simulink model "A1MODEL_Synthetic_Inv_Resp_delay"  (R2019a)
settings: Solver=VariableStepAuto  StartTime=0  StopTime=20  RelTol=1e-3
values from neighbouring files (symbols this model uses):
  c = 1    [calc_nadir.m]    (also in calc_variables_block.m; graph_freq_SI.m; graph_freq_SI_normal.m = 0; graph_freq_fpr.m)
  ci = 0    [calc_nadir.m]    (also in calc_variables_block.m; graph_freq_SI.m = 1; graph_freq_SI_normal.m = 1; graph_freq_fpr.m)
  d = 0.2    [calc_nadir.m]    (also in calc_variables_block.m = 0.001)
  E_load = 0    [calc_nadir.m]    (also in calc_variables_block.m; graph_freq_SI.m; graph_freq_SI_normal.m; graph_freq_fpr.m)
  F = data1(7)    [calc_nadir.m]    (also in calc_variables_block.m; graph_freq_SI.m; graph_freq_SI_normal.m; graph_freq_fpr.m)
  H = data1(9)    [calc_nadir.m]    (also in calc_variables_block.m; graph_freq_SI.m; graph_freq_SI_normal.m; graph_freq_fpr.m)
  H_wt = 4.37    [calc_nadir.m]    (also in calc_variables_block.m; graph_freq_SI.m; graph_freq_SI_normal.m; graph_freq_fpr.m)
  J = 3.56    [calc_nadir.m]    (also in calc_variables_block.m; graph_freq_SI.m; graph_freq_SI_normal.m; graph_freq_fpr.m)
  Ki = 10    [calc_nadir.m]    (also in calc_variables_block.m; graph_freq_SI.m; graph_freq_SI_normal.m; graph_freq_fpr.m)
  n_wt = P_re*share_wt/1.5    [calc_nadir.m]    (also in calc_variables_block.m; graph_freq_SI.m = P_wt/1.5; graph_freq_SI_normal.m = 0.666666666667; graph_freq_fpr.m)
  P_wt = P_re*share_wt    [calc_nadir.m]    (also in calc_variables_block.m; graph_freq_SI.m; graph_freq_SI_normal.m; graph_freq_fpr.m)
  R = 0.05    [calc_nadir.m]    (also in calc_variables_block.m; graph_freq_SI.m; graph_freq_SI_normal.m; graph_freq_fpr.m)
  Sb = data1(1)    [calc_nadir.m]    (also in calc_variables_block.m; graph_freq_SI.m; graph_freq_SI_normal.m; graph_freq_fpr.m)
  T_1 = data1(2)    [calc_nadir.m]    (also in calc_variables_block.m; graph_freq_SI.m; graph_freq_SI_normal.m; graph_freq_fpr.m)
  T_2 = data1(3)    [calc_nadir.m]    (also in calc_variables_block.m; graph_freq_SI.m; graph_freq_SI_normal.m; graph_freq_fpr.m)
  T_3 = data1(4)    [calc_nadir.m]    (also in calc_variables_block.m; graph_freq_SI.m; graph_freq_SI_normal.m; graph_freq_fpr.m)
  T_4 = data1(5)    [calc_nadir.m]    (also in calc_variables_block.m; graph_freq_SI.m; graph_freq_SI_normal.m; graph_freq_fpr.m)
  T_5 = data1(6)    [calc_nadir.m]    (also in calc_variables_block.m; graph_freq_SI.m; graph_freq_SI_normal.m; graph_freq_fpr.m)
  T_wt = 1    [calc_nadir.m]    (also in calc_variables_block.m; graph_freq_SI.m; graph_freq_SI_normal.m; graph_freq_fpr.m)
  un = 0.4    [calc_nadir.m]    (also in calc_variables_block.m; graph_freq_SI.m; graph_freq_SI_normal.m = 0.15; graph_freq_fpr.m = 0.25)
libraries: simulink x1
settings Model: Creator=estuser04  LastModifiedBy=Alejandro
settings DataIOCC: ReturnWorkspaceOutputs=off
settings DebuggingCC: ArithmeticOperatorsInVariantConditions=warning

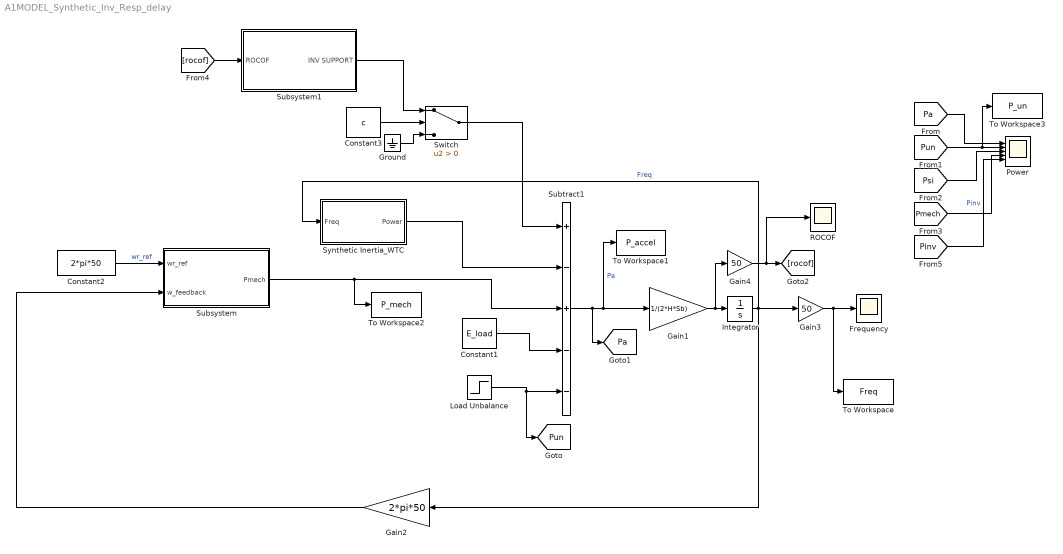
== system A1MODEL_Synthetic_Inv_Resp_delay ==
  Constant1 : Constant  Value=E_load
  Constant2 : Constant  Value=2*pi*50
  Constant3 : Constant  Value=c
  "Frequency " : Scope
  Gain1 : Gain  Gain=1/(2*H*Sb)
  Gain2 : Gain  Gain=2*pi*50
  Gain3 : Gain  Gain=50
  Gain4 : Gain  Gain=50
  Ground : Ground
  Integrator : Integrator  InitialCondition=1
  Load Unbalance : Step  Time=0  After=315*un  SampleTime=0
  Power : Scope  NumInputPorts=5
  ROCOF : Scope
  Subsystem : Subsystem
  Subsystem1 : Subsystem
  Subtract1 : Sum  Inputs=+-+--
  Switch : Switch  Criteria=u2 > Threshold
  "Synthetic Inertia_WTC " : Subsystem
  To Workspace : ToWorkspace  VariableName=Freq  SaveFormat=Timeseries  SampleTime=-1
  To Workspace1 : ToWorkspace  VariableName=P_accel  SaveFormat=Timeseries  SampleTime=-1
  To Workspace2 : ToWorkspace  VariableName=P_mech  SaveFormat=Timeseries  SampleTime=-1
  To Workspace3 : ToWorkspace  VariableName=P_un  SaveFormat=Timeseries  SampleTime=-1
  tag scope: Pa=global, Pun=global
  wires:
  Gain1/1 -> Gain4/1, Integrator/1
  Integrator/1 -> "Synthetic Inertia_WTC "/1(Freq), Gain3/1, Gain2/1  "Freq"
  Subtract1/1 -> [Pa], To Workspace1/1, Gain1/1  "Pa"
  Constant1/1 -> Subtract1/4
  Load Unbalance/1 -> Subtract1/5, [Pun]
  Gain3/1 -> To Workspace/1, "Frequency "/1
  Constant2/1 -> Subsystem/1(wr_ref)  "wr_ref"
  Gain2/1 -> Subsystem/2(w_feedback)
  Subsystem/1(Pmech) -> Subtract1/3, To Workspace2/1
  [Pa] -> Power/1
  [Pun] -> To Workspace3/1, Power/2
  [Psi] -> Power/3
  [Pmech] -> Power/4
  Switch/1 -> Subtract1/1
  Ground/1 -> Switch/3
  Constant3/1 -> Switch/2
  Gain4/1 -> ROCOF/1, [rocof]
  [rocof] -> Subsystem1/1(ROCOF)
  [Pinv] -> Power/5  "Pinv"
  "Synthetic Inertia_WTC "/1("Power ") -> Subtract1/2
  Subsystem1/1(INV SUPPORT) -> Switch/1

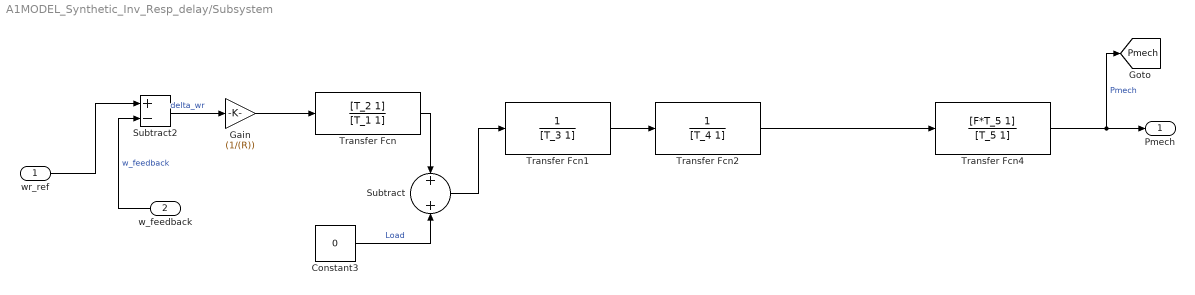
== system A1MODEL_Synthetic_Inv_Resp_delay/Subsystem ==
  wr_ref : Inport
  w_feedback : Inport  Port=2
  Constant3 : Constant  Value=0
  Gain : Gain  Gain=(1/(R))
  Subtract : Sum
  Subtract2 : Sum  Inputs=+-
  Transfer Fcn : TransferFcn  Numerator=[T_2 1]  Denominator=[T_1 1]
  Transfer Fcn1 : TransferFcn  Denominator=[T_3 1]
  Transfer Fcn2 : TransferFcn  Denominator=[T_4 1]
  Transfer Fcn4 : TransferFcn  Numerator=[F*T_5 1]  Denominator=[T_5 1]
  Pmech : Outport
  tag scope: Pmech=global
  wires:
  Constant3/1 -> Subtract/2  "Load"
  Transfer Fcn/1 -> Subtract/1
  Gain/1 -> Transfer Fcn/1
  Transfer Fcn2/1 -> Transfer Fcn4/1
  Subtract/1 -> Transfer Fcn1/1
  Subtract2/1 -> Gain/1  "delta_wr"
  w_feedback/1 -> Subtract2/2  "w_feedback"
  Transfer Fcn1/1 -> Transfer Fcn2/1
  wr_ref/1 -> Subtract2/1
  Transfer Fcn4/1 -> [Pmech], Pmech/1  "Pmech"

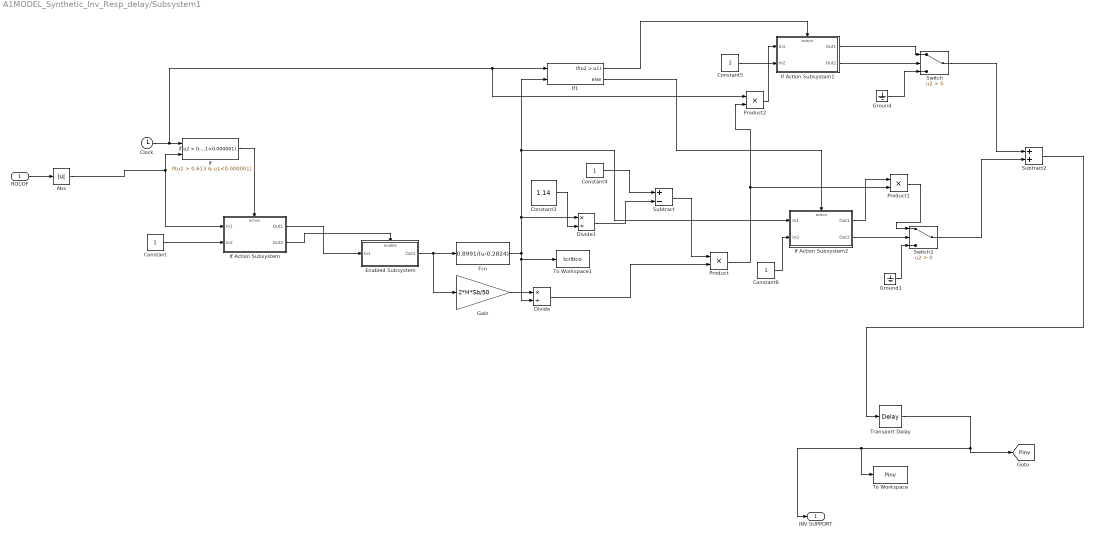
== system A1MODEL_Synthetic_Inv_Resp_delay/Subsystem1 ==
  ROCOF : Inport
  Abs : Abs  ZeroCross=off
  Clock : Clock
  Constant{,4..6} (4 alike) : Constant
  Constant3 : Constant  Value=1.14
  Divide : Product  Inputs=*/
  Divide1 : Product  Inputs=*/
  Enabled Subsystem : Subsystem  TreatAsAtomicUnit=on
  Fcn : Fcn  Expr=0.8991/(u-0.2824)
  Gain : Gain  Gain=2*H*Sb/50
  Ground : Ground
  Ground1 : Ground
  If : If  NumInputs=2  IfExpression=u2 > 0.613 & u1<0.000001  ShowElse=off
  If Action Subsystem : Subsystem  TreatAsAtomicUnit=on
  If Action Subsystem1 : Subsystem  TreatAsAtomicUnit=on
  If Action Subsystem2 : Subsystem  TreatAsAtomicUnit=on
  If1 : If  NumInputs=2  IfExpression=u2 > u1
  Product : Product
  Product1 : Product
  Product2 : Product
  Subtract : Sum  Inputs=+-
  Subtract2 : Sum
  Switch : Switch  Criteria=u2 > Threshold
  Switch1 : Switch  Criteria=u2 > Threshold
  To Workspace : ToWorkspace  VariableName=Pinv  SaveFormat=Timeseries  SampleTime=-1
  To Workspace1 : ToWorkspace  VariableName=tcritico  SaveFormat=Timeseries  SampleTime=-1
  Transport Delay : TransportDelay  DelayTime=d
  INV SUPPORT : Outport
  tag scope: Pinv=global
  wires:
  Switch1/1 -> Subtract2/2
  If Action Subsystem2/2(Out2) -> Switch1/2
  Divide/1 -> Product/2
  Product/1 -> Product1/2, Product2/2
  Constant4/1 -> Subtract/1
  Fcn/1 -> Divide/2, To Workspace1/1, If Action Subsystem2/1(In1), If1/2, Divide1/1
  If Action Subsystem/2(Out2) -> Enabled Subsystem/Enable
  Clock/1 -> Product2/1, If1/1, If/1
  Ground/1 -> Switch/3
  Divide1/1 -> Subtract/2
  Constant3/1 -> Divide1/2
  Enabled Subsystem/1(Out1) -> Gain/1, Fcn/1
  If Action Subsystem/1(Out1) -> Enabled Subsystem/1(In1)
  Subtract/1 -> Product/1
  If Action Subsystem1/2(Out2) -> Switch/2
  If1/1 -> If Action Subsystem1/Action
  Subtract2/1 -> Transport Delay/1
  Gain/1 -> Divide/1
  Ground1/1 -> Switch1/3
  If Action Subsystem2/1(Out1) -> Product1/1
  ROCOF/1 -> Abs/1
  Product1/1 -> Switch1/1
  If Action Subsystem1/1(Out1) -> Switch/1
  Constant6/1 -> If Action Subsystem2/2(In2)
  Constant5/1 -> If Action Subsystem1/2(In2)
  Switch/1 -> Subtract2/1
  Constant/1 -> If Action Subsystem/2(In2)
  Abs/1 -> If Action Subsystem/1(In1), If/2
  If1/2 -> If Action Subsystem2/Action
  Product2/1 -> If Action Subsystem1/1(In1)
  Transport Delay/1 -> [Pinv], To Workspace/1, INV SUPPORT/1
  If/1 -> If Action Subsystem/Action

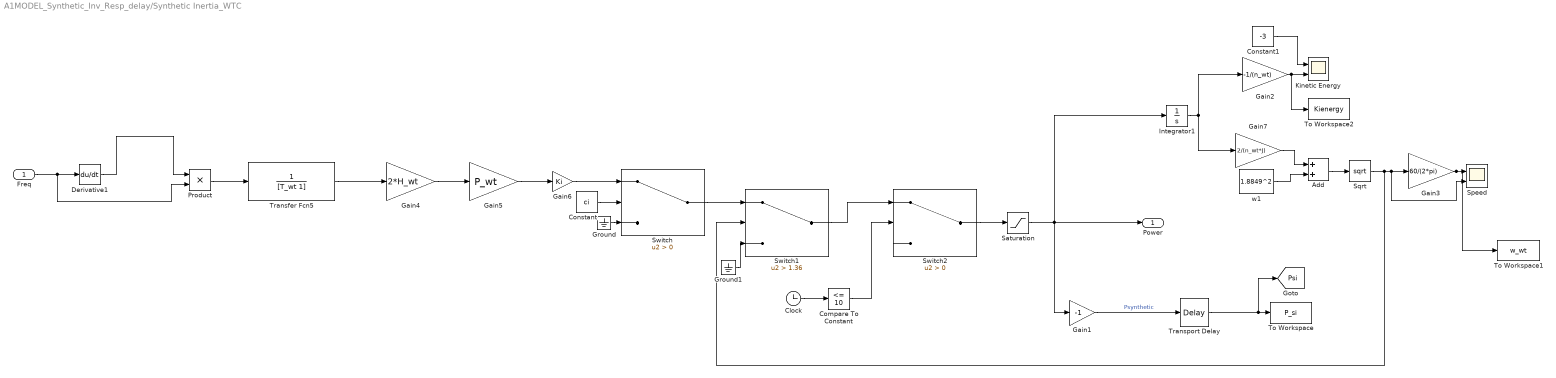
== system A1MODEL_Synthetic_Inv_Resp_delay/Synthetic Inertia_WTC  ==
  Freq : Inport
  Add : Sum
  Clock : Clock
  Compare To Constant : simulink/Logic and Bit Operations/Compare To Constant  relop=<=  const=10  OutDataTypeStr=boolean
  Constant : Constant  Value=ci
  Constant1 : Constant  Value=-3
  Derivative1 : Derivative
  Gain1 : Gain  Gain=-1
  Gain2 : Gain  Gain=-1/(n_wt)
  Gain3 : Gain  Gain=60/(2*pi)
  Gain4 : Gain  Gain=2*H_wt
  Gain5 : Gain  Gain=P_wt
  Gain6 : Gain  Gain=Ki
  Gain7 : Gain  Gain=2/(n_wt*J)
  Ground : Ground
  Ground1 : Ground
  Integrator1 : Integrator
  "Kinetic Energy " : Scope  NumInputPorts=2
  Product : Product
  Saturation : Saturate  UpperLimit=0  LowerLimit=-P_wt*0.10
  "Speed " : Scope  NumInputPorts=2
  Sqrt : Sqrt  SaturateOnIntegerOverflow=on
  Switch : Switch  Criteria=u2 > Threshold
  Switch1 : Switch  Criteria=u2 > Threshold  Threshold=1.36
  Switch2 : Switch  Criteria=u2 > Threshold
  To Workspace : ToWorkspace  VariableName=P_si  SaveFormat=Timeseries  SampleTime=-1
  To Workspace1 : ToWorkspace  VariableName=w_wt  SaveFormat=Timeseries  SampleTime=-1
  To Workspace2 : ToWorkspace  VariableName=Kienergy  SaveFormat=Timeseries  SampleTime=-1
  Transfer Fcn5 : TransferFcn  Denominator=[T_wt 1]
  Transport Delay : TransportDelay  DelayTime=d
  w1 : Constant  Value=1.8849^2
  "Power " : Outport
  tag scope: Psi=global
  wires:
  Gain5/1 -> Gain6/1
  Switch/1 -> Switch1/1
  Gain7/1 -> Add/1
  Gain4/1 -> Gain5/1
  Add/1 -> Sqrt/1
  Freq/1 -> Product/2, Derivative1/1
  w1/1 -> Add/2
  Product/1 -> Transfer Fcn5/1
  Transfer Fcn5/1 -> Gain4/1
  Constant/1 -> Switch/2
  Integrator1/1 -> Gain7/1, Gain2/1
  Gain6/1 -> Switch/1
  Ground/1 -> Switch/3
  Gain1/1 -> Transport Delay/1  "Psynthetic"
  Switch1/1 -> Switch2/1
  Sqrt/1 -> Switch1/2, "Speed "/2, Gain3/1
  Ground1/1 -> Switch1/3
  Gain2/1 -> To Workspace2/1, "Kinetic Energy "/2
  Constant1/1 -> "Kinetic Energy "/1
  Saturation/1 -> "Power "/1, Gain1/1, Integrator1/1
  Derivative1/1 -> Product/1
  Gain3/1 -> To Workspace1/1, "Speed "/1
  Clock/1 -> Compare To Constant/1
  Compare To Constant/1 -> Switch2/2
  Switch2/1 -> Saturation/1
  Transport Delay/1 -> [Psi], To Workspace/1

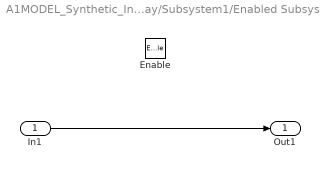
== system A1MODEL_Synthetic_Inv_Resp_delay/Subsystem1/Enabled Subsystem ==
  In1 : Inport
  Enable : EnablePort
  Out1 : Outport
  wires:
  In1/1 -> Out1/1

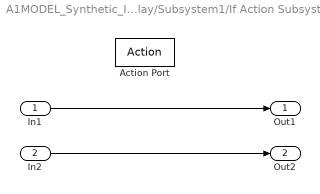
== system A1MODEL_Synthetic_Inv_Resp_delay/Subsystem1/If Action Subsystem ==
  In1 : Inport
  In2 : Inport  Port=2
  Action Port : ActionPort  ActionPortLabel=if(u2 > 0.613 & u1<0.000001)
  Out1 : Outport
  Out2 : Outport  Port=2
  wires:
  In1/1 -> Out1/1
  In2/1 -> Out2/1

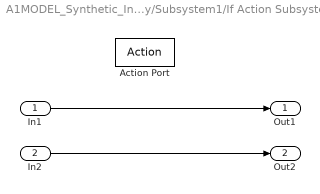
== system A1MODEL_Synthetic_Inv_Resp_delay/Subsystem1/If Action Subsystem1 ==
  In1 : Inport
  In2 : Inport  Port=2
  Action Port : ActionPort  ActionPortLabel=if(u2 > u1)
  Out1 : Outport  OutputWhenDisabled=reset  InitialOutput=0
  Out2 : Outport  Port=2  OutputWhenDisabled=reset  InitialOutput=0
  wires:
  In1/1 -> Out1/1
  In2/1 -> Out2/1

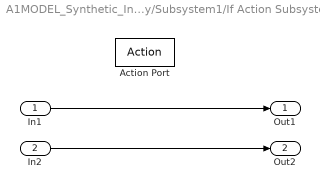
== system A1MODEL_Synthetic_Inv_Resp_delay/Subsystem1/If Action Subsystem2 ==
  In1 : Inport
  In2 : Inport  Port=2
  Action Port : ActionPort  ActionPortLabel=else
  Out1 : Outport  OutputWhenDisabled=reset  InitialOutput=0
  Out2 : Outport  Port=2  InitialOutput=0
  wires:
  In1/1 -> Out1/1
  In2/1 -> Out2/1
